simulink model "banc_essai_non_lineaire"  (R2021a)
settings: Solver=ode45  StartTime=0.0  StopTime=tfin  FixedStep=0.001  RelTol=1e-09  EnableMultiTasking=on
values from neighbouring files (symbols this model uses):
  Pzeq = .015    (= 0.015)    [main_non_lineaire.m]
undefined symbols (not defined in the file or in its folder): ae0, ae1, ae2, ae3, as0, as1, as2, as3, be1, g, Jx, Jy, LA, LB, LC, mSeff, mSg, mtot, RA, RB, RC, Vmax, XA, XB, XC, XD, XE, XF, YA, YB, YC, YD, YE, YF
settings Model: PacingRate=0.160000  Creator=delafontaine  LastModifiedBy=User
settings SolverCC: AlgebraicLoopSolver=LineSearch
settings DataIOCC: LimitDataPoints=on  SaveFormat=Array  SignalLoggingSaveFormat=ModelDataLogs  ReturnWorkspaceOutputs=off
settings OptimizationCC: LifeSpan=inf
settings DebuggingCC: UnderspecifiedInitializationDetection=Classic  MergeDetectMultiDrivingBlocksExec=none  MultiTaskDSMMsg=warning  MultiTaskCondExecSysMsg=none  SFUnexpectedBacktrackingDiag=warning  SFNoUnconditionalDefaultTransitionDiag=warning  SFExecutionAtInitializationDiag=none  SFMachineParentedDataDiag=warning  ArithmeticOperatorsInVariantConditions=warning
settings HardwareCC: ProdBitPerPointer=32  ProdBitPerSizeT=32  ProdBitPerPtrDiffT=32  ProdLargestAtomicFloat=None  ProdIntDivRoundTo=Undefined  ProdEndianess=Unspecified  ProdWordSize=32  ProdHWDeviceType=32-bit Generic
settings ModelReferenceCC: PropagateSignalLabelsOutOfModel=off
settings SFSimCC: SimUseLocalCustomCode=off  CustomCodeUndefinedFunction=UseInterfaceOnly
settings RTWCC: RTWUseLocalCustomCode=off
settings CodeAppCC: StateflowObjectComments=on
settings GRTTargetCC: TargetLangStandard=C89/C90 (ANSI)
settings ConfigComp: CovMetricSettings=dw  CovSaveCumulativeToWorkspaceVar=on  CovSaveSingleToWorkspaceVar=on  CovExternalEMLEnable=off  CovSFcnEnable=off

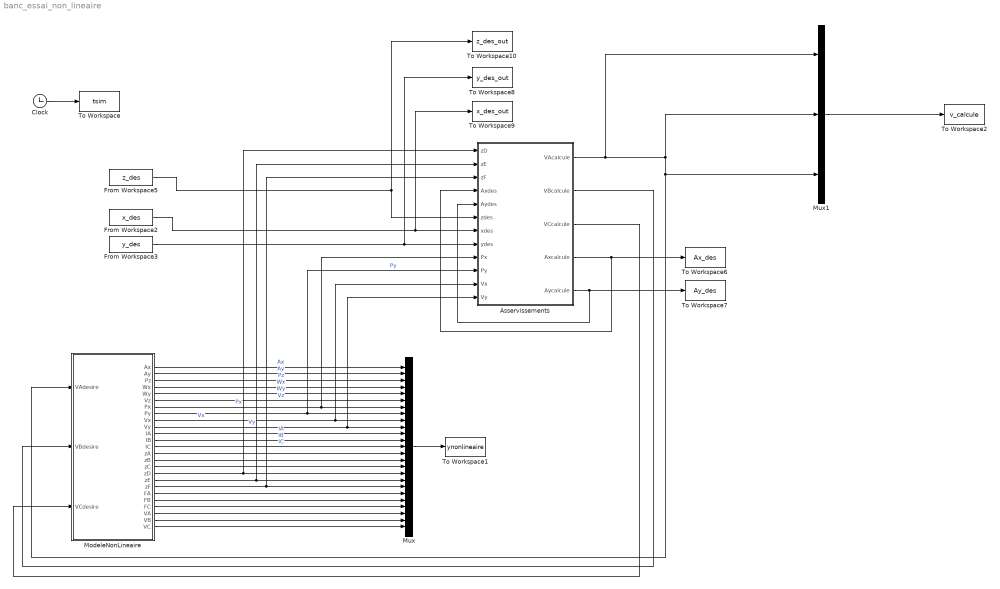
== system banc_essai_non_lineaire ==
  Asservissements : Subsystem
      mask help: Simulink:masks:GenSFuncDesc_MD
      mask Help: eval('feval(''rtwprivate'',''rtwhelpview'',''rtw_sfcn_block'')');
  Clock : Clock
  From Workspace2 : FromWorkspace  VariableName=x_des  Interpolate=off  OutputAfterFinalValue=Holding final value
  From Workspace3 : FromWorkspace  VariableName=y_des  Interpolate=off  OutputAfterFinalValue=Holding final value
  From Workspace5 : FromWorkspace  VariableName=z_des  Interpolate=off  OutputAfterFinalValue=Holding final value
  ModeleNonLineaire : Subsystem
      mask help: Simulink:masks:GenSFuncDesc_MD
      mask Help: eval('feval(''rtwprivate'',''rtwhelpview'',''rtw_sfcn_block'')');
  Mux : Mux  Inputs=25
  Mux1 : Mux  Inputs=3
  To Workspace : ToWorkspace  VariableName=tsim  SampleTime=-1
  To Workspace1 : ToWorkspace  VariableName=ynonlineaire  SampleTime=-1
  To Workspace10 : ToWorkspace  VariableName=z_des_out  SampleTime=-1
  To Workspace2 : ToWorkspace  VariableName=v_calcule  SampleTime=-1
  To Workspace6 : ToWorkspace  VariableName=Ax_des  SampleTime=-1
  To Workspace7 : ToWorkspace  VariableName=Ay_des  SampleTime=-1
  To Workspace8 : ToWorkspace  VariableName=y_des_out  SampleTime=-1
  To Workspace9 : ToWorkspace  VariableName=x_des_out  SampleTime=-1
  wires:
  Mux/1 -> To Workspace1/1
  Clock/1 -> To Workspace/1
  From Workspace5/1 -> Asservissements/6(zdes), To Workspace10/1
  ModeleNonLineaire/1(Ax) -> Mux/1  "Ax"
  ModeleNonLineaire/2(Ay) -> Mux/2  "Ay"
  ModeleNonLineaire/3(Pz) -> Mux/3  "Pz"
  ModeleNonLineaire/4(Wx) -> Mux/4  "Wx"
  ModeleNonLineaire/5(Wy) -> Mux/5  "Wy"
  ModeleNonLineaire/6(Vz) -> Mux/6  "Vz"
  ModeleNonLineaire/7(Px) -> Asservissements/9(Px), Mux/7  "Px"
  ModeleNonLineaire/8(Py) -> Asservissements/10(Py), Mux/8  "Py"
  ModeleNonLineaire/9(Vx) -> Asservissements/11(Vx), Mux/9  "Vx"
  ModeleNonLineaire/10(Vy) -> Asservissements/12(Vy), Mux/10  "Vy"
  ModeleNonLineaire/11(IA) -> Mux/11  "IA"
  ModeleNonLineaire/12(IB) -> Mux/12  "IB"
  ModeleNonLineaire/13(IC) -> Mux/13  "IC"
  From Workspace3/1 -> Asservissements/8(ydes), To Workspace8/1
  From Workspace2/1 -> Asservissements/7(xdes), To Workspace9/1
  ModeleNonLineaire/20(FA) -> Mux/20
  ModeleNonLineaire/21(FB) -> Mux/21
  ModeleNonLineaire/22(FC) -> Mux/22
  ModeleNonLineaire/23(VA) -> Mux/23
  ModeleNonLineaire/24(VB) -> Mux/24
  ModeleNonLineaire/25(VC) -> Mux/25
  Asservissements/4(Axcalcule) -> Asservissements/4(Axdes), To Workspace6/1
  Asservissements/5(Aycalcule) -> Asservissements/5(Aydes), To Workspace7/1
  Asservissements/1(VAcalcule) -> Mux1/1, Mux1/2, ModeleNonLineaire/1(VAdesire), Mux1/3
  Asservissements/2(VBcalcule) -> ModeleNonLineaire/2(VBdesire)
  Asservissements/3(VCcalcule) -> ModeleNonLineaire/3(VCdesire)
  ModeleNonLineaire/16(zC) -> Mux/16
  ModeleNonLineaire/17(zD) -> Asservissements/1(zD), Mux/17
  ModeleNonLineaire/18(zE) -> Asservissements/2(zE), Mux/18
  ModeleNonLineaire/19(zF) -> Asservissements/3(zF), Mux/19
  ModeleNonLineaire/14(zA) -> Mux/14
  ModeleNonLineaire/15(zB) -> Mux/15
  Mux1/1 -> To Workspace2/1

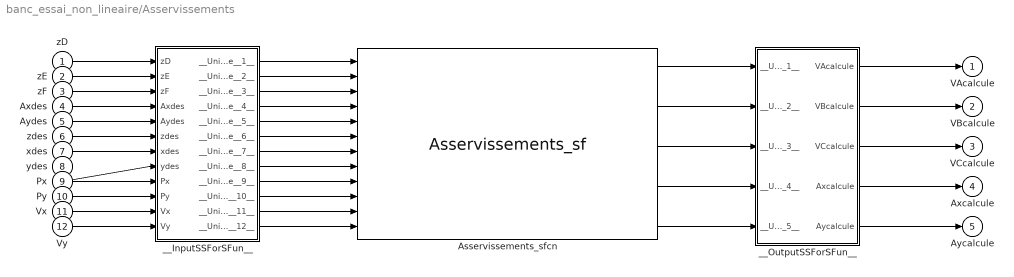
== system banc_essai_non_lineaire/Asservissements ==
  zD : Inport
  zE : Inport  Port=2
  zF : Inport  Port=3
  Axdes : Inport  Port=4
  Aydes : Inport  Port=5
  zdes : Inport  Port=6
  xdes : Inport  Port=7
  ydes : Inport  Port=8
  Px : Inport  Port=9
  Py : Inport  Port=10
  Vx : Inport  Port=11
  Vy : Inport  Port=12
  Asservissements_sfcn : S-Function  FunctionName=Asservissements_sf  SFunctionModules=""  SFunctionDeploymentMode=off  EnableBusSupport=off  mask{rtw_sf_name=Asservissements_sf, showVar=off}
      mask prompts: rtw_sf_name "Simulink:masks:GenSFuncName_MP"; showVar "Simulink:masks:GenSFuncShowModuleList_MP"
      mask help: Simulink:masks:GenSFuncDesc_MD
      mask init:
      | displist = '';
      | if ~strcmp(get_param(gcb, 'FunctionName'), rtw_sf_name);
      |   set_param(gcb, 'FunctionName', rtw_sf_name);
      | end
      | % Check if we are generating code
      | rtw_mode = false;
      | if strcmpi(get_param(bdroot(gcb),'SimulationStatus'),'Initializing')
      | 	rtw_mode = strcmpi(get_param(bdroot(gcb),'BuildingRTWCode'),'on') && ...
      | 		~strcmpi(get_param(bdroot(gcb),'TargetStyle'),'SimulationTarget');
      | end
      | if showVar || rtw_mode
      | 	if exist('rtwsfunc') == 2 | exist('rtwsfunc') == 6
      | 		tmplist = rtwsfunc(rtw_sf_name,gcb);
      | 		tmplist = DAStudio.message('Simulink:masks:GenSFuncListOfModules_IC', tmplist);
      | 	elseif showVar
      | 		tmplist1 = DAStudio.message('Simulink:masks:GenSFuncListOfModules_IC', '');
      |         tmplist2 = DAStudio.message('Simulink:masks:GenSFuncNotLicensed_IC');
      |         tmplist = [tmplist1 tmplist2];
      |  	end
      | end
      | if showVar
      |   displist = tmplist;
      | end
      settings: CopyFcn=|
      | if ~strcmp(get_param(gcb,'Linkstatus'),'none') && ...
      | ~strcmp(get_param(gcb,'Linkstatus'),'implicit')
      |   set_param(gcb,'LinkStatus','none');
      | end
      mask Help: eval('feval(''rtwprivate'',''rtwhelpview'',''rtw_sfcn_block'')');
      mask Display:
      | port_label('input',1,'zD');
      | port_label('input',2,'zE');
      | port_label('input',3,'zF');
      | port_label('input',4,'Axdes');
      | port_label('input',5,'Aydes');
      | port_label('input',6,'zdes');
      | port_label('input',7,'xdes');
      | port_label('input',8,'ydes');
      | port_label('input',9,'Px');
      | port_label('input',10,'Py');
      | port_label('input',11,'Vx');
      | port_label('input',12,'Vy');
      | port_label('output',1,'VAcalcule');
      | port_label('output',2,'VBcalcule');
      | port_label('output',3,'VCcalcule');
      | port_label('output',4,'Axcalcule');
      | port_label('output',5,'Aycalcule');
  __InputSSForSFun__ : Subsystem
  __OutputSSForSFun__ : Subsystem
  VAcalcule : Outport
  VBcalcule : Outport  Port=2
  VCcalcule : Outport  Port=3
  Axcalcule : Outport  Port=4
  Aycalcule : Outport  Port=5
  wires:
  zD/1 -> __InputSSForSFun__/1(zD)
  zE/1 -> __InputSSForSFun__/2(zE)
  zF/1 -> __InputSSForSFun__/3(zF)
  Axdes/1 -> __InputSSForSFun__/4(Axdes)
  Aydes/1 -> __InputSSForSFun__/5(Aydes)
  zdes/1 -> __InputSSForSFun__/6(zdes)
  xdes/1 -> __InputSSForSFun__/7(xdes)
  ydes/1 -> __InputSSForSFun__/8(ydes)
  Px/1 -> __InputSSForSFun__/9(Px)
  Py/1 -> __InputSSForSFun__/10(Py)
  Vx/1 -> __InputSSForSFun__/11(Vx)
  Vy/1 -> __InputSSForSFun__/12(Vy)
  __InputSSForSFun__/1(__UniqueOutportName__1__) -> Asservissements_sfcn/1
  __InputSSForSFun__/2(__UniqueOutportName__2__) -> Asservissements_sfcn/2
  __InputSSForSFun__/3(__UniqueOutportName__3__) -> Asservissements_sfcn/3
  __InputSSForSFun__/4(__UniqueOutportName__4__) -> Asservissements_sfcn/4
  __InputSSForSFun__/5(__UniqueOutportName__5__) -> Asservissements_sfcn/5
  __InputSSForSFun__/6(__UniqueOutportName__6__) -> Asservissements_sfcn/6
  __InputSSForSFun__/7(__UniqueOutportName__7__) -> Asservissements_sfcn/7
  __InputSSForSFun__/8(__UniqueOutportName__8__) -> Asservissements_sfcn/8
  __InputSSForSFun__/9(__UniqueOutportName__9__) -> Asservissements_sfcn/9
  __InputSSForSFun__/10(__UniqueOutportName__10__) -> Asservissements_sfcn/10
  __InputSSForSFun__/11(__UniqueOutportName__11__) -> Asservissements_sfcn/11
  __InputSSForSFun__/12(__UniqueOutportName__12__) -> Asservissements_sfcn/12
  Asservissements_sfcn/1 -> __OutputSSForSFun__/1(__UniqueInportName__1__)
  Asservissements_sfcn/2 -> __OutputSSForSFun__/2(__UniqueInportName__2__)
  Asservissements_sfcn/3 -> __OutputSSForSFun__/3(__UniqueInportName__3__)
  Asservissements_sfcn/4 -> __OutputSSForSFun__/4(__UniqueInportName__4__)
  Asservissements_sfcn/5 -> __OutputSSForSFun__/5(__UniqueInportName__5__)
  __OutputSSForSFun__/1(VAcalcule) -> VAcalcule/1
  __OutputSSForSFun__/2(VBcalcule) -> VBcalcule/1
  __OutputSSForSFun__/3(VCcalcule) -> VCcalcule/1
  __OutputSSForSFun__/4(Axcalcule) -> Axcalcule/1
  __OutputSSForSFun__/5(Aycalcule) -> Aycalcule/1

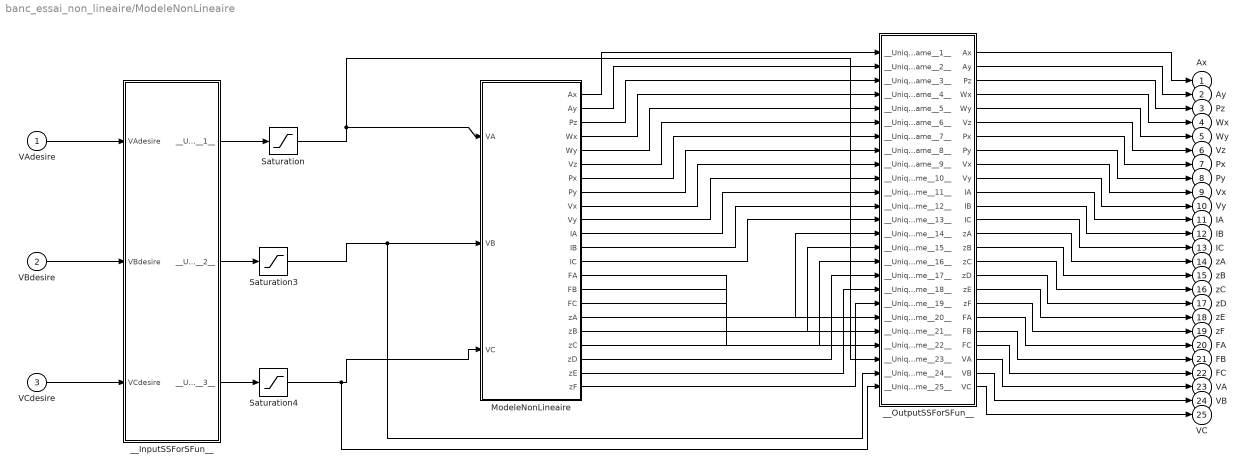
== system banc_essai_non_lineaire/ModeleNonLineaire ==
  VAdesire : Inport
  VBdesire : Inport  Port=2
  VCdesire : Inport  Port=3
  ModeleNonLineaire : Subsystem
  Saturation : Saturate  UpperLimit=0  LowerLimit=-Vmax
  Saturation3 : Saturate  UpperLimit=0  LowerLimit=-Vmax
  Saturation4 : Saturate  UpperLimit=0  LowerLimit=-Vmax
  __InputSSForSFun__ : Subsystem
  __OutputSSForSFun__ : Subsystem
  Ax : Outport
  Ay : Outport  Port=2
  Pz : Outport  Port=3
  Wx : Outport  Port=4
  Wy : Outport  Port=5
  Vz : Outport  Port=6
  Px : Outport  Port=7
  Py : Outport  Port=8
  Vx : Outport  Port=9
  Vy : Outport  Port=10
  IA : Outport  Port=11
  IB : Outport  Port=12
  IC : Outport  Port=13
  zA : Outport  Port=14
  zB : Outport  Port=15
  zC : Outport  Port=16
  zD : Outport  Port=17
  zE : Outport  Port=18
  zF : Outport  Port=19
  FA : Outport  Port=20
  FB : Outport  Port=21
  FC : Outport  Port=22
  VA : Outport  Port=23
  VB : Outport  Port=24
  VC : Outport  Port=25
  wires:
  VAdesire/1 -> __InputSSForSFun__/1(VAdesire)
  VBdesire/1 -> __InputSSForSFun__/2(VBdesire)
  VCdesire/1 -> __InputSSForSFun__/3(VCdesire)
  __InputSSForSFun__/2(__UniqueOutportName__2__) -> Saturation3/1
  __InputSSForSFun__/3(__UniqueOutportName__3__) -> Saturation4/1
  ModeleNonLineaire/1(Ax) -> __OutputSSForSFun__/1(__UniqueInportName__1__)
  ModeleNonLineaire/2(Ay) -> __OutputSSForSFun__/2(__UniqueInportName__2__)
  ModeleNonLineaire/3(Pz) -> __OutputSSForSFun__/3(__UniqueInportName__3__)
  ModeleNonLineaire/4(Wx) -> __OutputSSForSFun__/4(__UniqueInportName__4__)
  ModeleNonLineaire/5(Wy) -> __OutputSSForSFun__/5(__UniqueInportName__5__)
  ModeleNonLineaire/6(Vz) -> __OutputSSForSFun__/6(__UniqueInportName__6__)
  ModeleNonLineaire/7(Px) -> __OutputSSForSFun__/7(__UniqueInportName__7__)
  ModeleNonLineaire/8(Py) -> __OutputSSForSFun__/8(__UniqueInportName__8__)
  ModeleNonLineaire/9(Vx) -> __OutputSSForSFun__/9(__UniqueInportName__9__)
  ModeleNonLineaire/10(Vy) -> __OutputSSForSFun__/10(__UniqueInportName__10__)
  ModeleNonLineaire/11(IA) -> __OutputSSForSFun__/11(__UniqueInportName__11__)
  ModeleNonLineaire/12(IB) -> __OutputSSForSFun__/12(__UniqueInportName__12__)
  ModeleNonLineaire/13(IC) -> __OutputSSForSFun__/13(__UniqueInportName__13__)
  __OutputSSForSFun__/1(Ax) -> Ax/1
  __OutputSSForSFun__/2(Ay) -> Ay/1
  __OutputSSForSFun__/3(Pz) -> Pz/1
  __OutputSSForSFun__/4(Wx) -> Wx/1
  __OutputSSForSFun__/5(Wy) -> Wy/1
  __OutputSSForSFun__/6(Vz) -> Vz/1
  __OutputSSForSFun__/7(Px) -> Px/1
  __OutputSSForSFun__/8(Py) -> Py/1
  __OutputSSForSFun__/9(Vx) -> Vx/1
  __OutputSSForSFun__/10(Vy) -> Vy/1
  __OutputSSForSFun__/11(IA) -> IA/1
  __OutputSSForSFun__/12(IB) -> IB/1
  __OutputSSForSFun__/13(IC) -> IC/1
  __OutputSSForSFun__/14(zA) -> zA/1
  __OutputSSForSFun__/15(zB) -> zB/1
  __OutputSSForSFun__/16(zC) -> zC/1
  __OutputSSForSFun__/17(zD) -> zD/1
  __OutputSSForSFun__/18(zE) -> zE/1
  __OutputSSForSFun__/19(zF) -> zF/1
  __OutputSSForSFun__/20(FA) -> FA/1
  __OutputSSForSFun__/21(FB) -> FB/1
  __OutputSSForSFun__/22(FC) -> FC/1
  __OutputSSForSFun__/23(VA) -> VA/1
  __OutputSSForSFun__/24(VB) -> VB/1
  __OutputSSForSFun__/25(VC) -> VC/1
  ModeleNonLineaire/14(FA) -> __OutputSSForSFun__/20(__UniqueInportName__20__)
  ModeleNonLineaire/15(FB) -> __OutputSSForSFun__/21(__UniqueInportName__21__)
  ModeleNonLineaire/16(FC) -> __OutputSSForSFun__/22(__UniqueInportName__22__)
  ModeleNonLineaire/17(zA) -> __OutputSSForSFun__/14(__UniqueInportName__14__)
  ModeleNonLineaire/18(zB) -> __OutputSSForSFun__/15(__UniqueInportName__15__)
  ModeleNonLineaire/19(zC) -> __OutputSSForSFun__/16(__UniqueInportName__16__)
  ModeleNonLineaire/20(zD) -> __OutputSSForSFun__/17(__UniqueInportName__17__)
  ModeleNonLineaire/21(zE) -> __OutputSSForSFun__/18(__UniqueInportName__18__)
  ModeleNonLineaire/22(zF) -> __OutputSSForSFun__/19(__UniqueInportName__19__)
  __InputSSForSFun__/1(__UniqueOutportName__1__) -> Saturation/1
  Saturation3/1 -> ModeleNonLineaire/2(VB), __OutputSSForSFun__/24(__UniqueInportName__24__)
  Saturation4/1 -> ModeleNonLineaire/3(VC), __OutputSSForSFun__/25(__UniqueInportName__25__)
  Saturation/1 -> ModeleNonLineaire/1(VA), __OutputSSForSFun__/23(__UniqueInportName__23__)

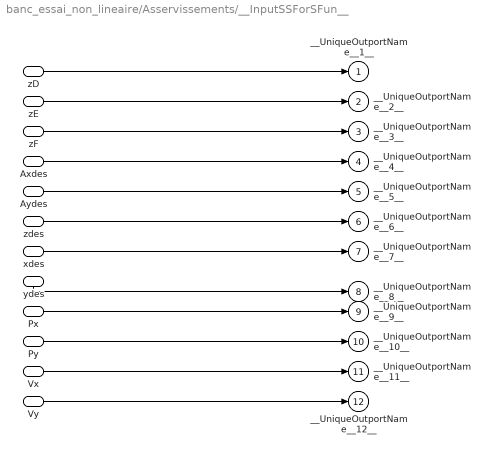
== system banc_essai_non_lineaire/Asservissements/__InputSSForSFun__ ==
  zD : Inport
  zE : Inport  Port=2
  zF : Inport  Port=3
  Axdes : Inport  Port=4
  Aydes : Inport  Port=5
  zdes : Inport  Port=6
  xdes : Inport  Port=7
  ydes : Inport  Port=8
  Px : Inport  Port=9
  Py : Inport  Port=10
  Vx : Inport  Port=11
  Vy : Inport  Port=12
  __UniqueOutportName__1__ : Outport
  __UniqueOutportName__2__ : Outport  Port=2
  __UniqueOutportName__3__ : Outport  Port=3
  __UniqueOutportName__4__ : Outport  Port=4
  __UniqueOutportName__5__ : Outport  Port=5
  __UniqueOutportName__6__ : Outport  Port=6
  __UniqueOutportName__7__ : Outport  Port=7
  __UniqueOutportName__8__ : Outport  Port=8
  __UniqueOutportName__9__ : Outport  Port=9
  __UniqueOutportName__10__ : Outport  Port=10
  __UniqueOutportName__11__ : Outport  Port=11
  __UniqueOutportName__12__ : Outport  Port=12
  wires:
  zD/1 -> __UniqueOutportName__1__/1
  zE/1 -> __UniqueOutportName__2__/1
  zF/1 -> __UniqueOutportName__3__/1
  Axdes/1 -> __UniqueOutportName__4__/1
  Aydes/1 -> __UniqueOutportName__5__/1
  zdes/1 -> __UniqueOutportName__6__/1
  xdes/1 -> __UniqueOutportName__7__/1
  ydes/1 -> __UniqueOutportName__8__/1
  Px/1 -> __UniqueOutportName__9__/1
  Py/1 -> __UniqueOutportName__10__/1
  Vx/1 -> __UniqueOutportName__11__/1
  Vy/1 -> __UniqueOutportName__12__/1

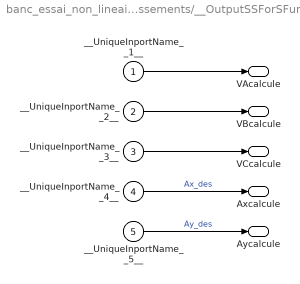
== system banc_essai_non_lineaire/Asservissements/__OutputSSForSFun__ ==
  __UniqueInportName__1__ : Inport
  __UniqueInportName__2__ : Inport  Port=2
  __UniqueInportName__3__ : Inport  Port=3
  __UniqueInportName__4__ : Inport  Port=4
  __UniqueInportName__5__ : Inport  Port=5
  VAcalcule : Outport
  VBcalcule : Outport  Port=2
  VCcalcule : Outport  Port=3
  Axcalcule : Outport  Port=4
  Aycalcule : Outport  Port=5
  wires:
  __UniqueInportName__1__/1 -> VAcalcule/1
  __UniqueInportName__2__/1 -> VBcalcule/1
  __UniqueInportName__3__/1 -> VCcalcule/1
  __UniqueInportName__4__/1 -> Axcalcule/1  "Ax_des"
  __UniqueInportName__5__/1 -> Aycalcule/1  "Ay_des"

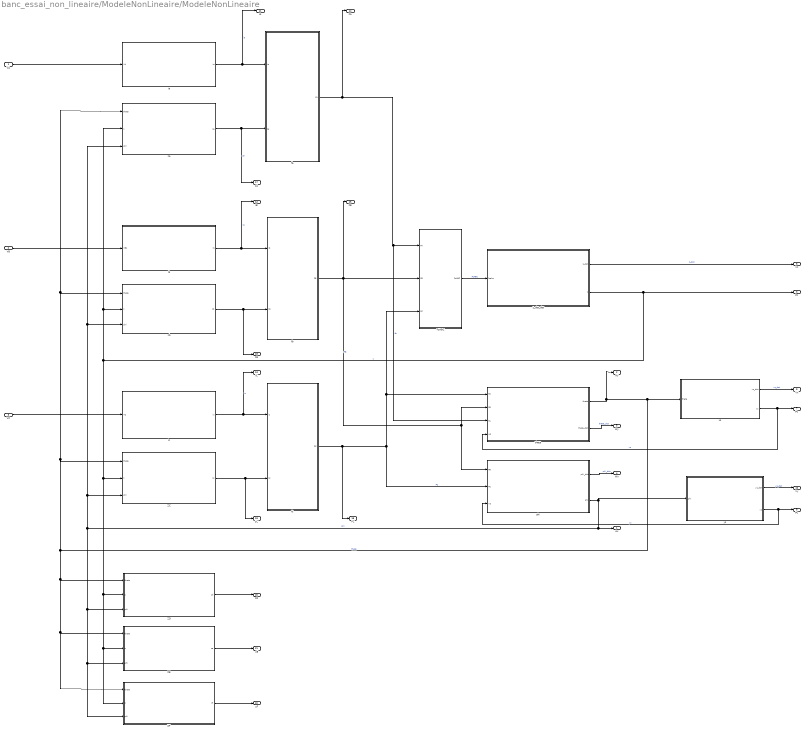
== system banc_essai_non_lineaire/ModeleNonLineaire/ModeleNonLineaire ==
  VA : Inport
  VB : Inport  Port=2
  VC : Inport  Port=3
  FzABC : Subsystem
  ZC : Subsystem
  ZD : Subsystem
  ZE : Subsystem
  ZF : Subsystem
  fa : Subsystem
  fb : Subsystem
  fc : Subsystem
  ia : Subsystem
  ib : Subsystem
  ic : Subsystem
  phi : Subsystem
  theta : Subsystem
  xs : Subsystem
  ys : Subsystem
  z_dot_dot : Subsystem
  za : Subsystem
  zb : Subsystem
  Ax : Outport
  Ay : Outport  Port=2
  Pz : Outport  Port=3
  Wx : Outport  Port=4
  Wy : Outport  Port=5
  Vz : Outport  Port=6
  Px : Outport  Port=7
  Py : Outport  Port=8
  Vx : Outport  Port=9
  Vy : Outport  Port=10
  IA : Outport  Port=11
  IB : Outport  Port=12
  IC : Outport  Port=13
  FA : Outport  Port=14
  FB : Outport  Port=15
  FC : Outport  Port=16
  zA : Outport  Port=17
  zB : Outport  Port=18
  zC : Outport  Port=19
  zD : Outport  Port=20
  zE : Outport  Port=21
  zF : Outport  Port=22
  wires:
  ia/1(ia) -> fa/1(ia), IA/1  "ia"
  ic/1(ic) -> IC/1, fc/1(ic)  "ic"
  phi/2(phi) -> ys/1(phi), Ax/1, za/3(phi), zb/3(phi), ZC/3(phi), ZD/3(phi), ZF/3(phi), ZE/3(phi)  "phi"
  theta/1(theta) -> xs/1(theta), ZD/1(theta), ZF/1(theta), ZE/1(theta), za/1(theta), zb/1(theta), ZC/1(theta), Ay/1  "theta"
  fa/1(FA) -> theta/3(FA), FzABC/1(FA), FA/1  "fa"
  fb/1(FB) -> FzABC/2(FB), phi/1(FB), theta/2(FB), FB/1  "FB"
  fc/1(FC) -> FC/1, phi/2(FC), FzABC/3(FC), theta/1(FC)  "FC"
  ZC/1(zc) -> zC/1, fc/2(zc)
  zb/1(zb) -> zB/1, fb/2(zb)
  ib/1(ib) -> fb/1(ib), IB/1  "ib"
  FzABC/1(FzABC) -> z_dot_dot/1(fzabc)  "FzABC"
  za/1(za) -> zA/1, fa/2(za)  "za"
  theta/2(theta_dot) -> Wy/1  "theta_dot"
  xs/1(xs_dot) -> Vx/1  "xs_dot"
  z_dot_dot/2(z) -> za/2(z), zb/2(z), ZD/2(z), ZF/2(z), ZE/2(z), ZC/2(z), Pz/1  "z"
  phi/1(phi_dot) -> Wx/1  "phi_dot"
  ys/2(ys) -> phi/3(YS), Py/1  "ys"
  VB/1 -> ib/1(VB1)
  z_dot_dot/1(z_dot) -> Vz/1  "z_dot"
  xs/2(xs) -> theta/4(XS), Px/1  "xs"
  ys/1(ys_dot) -> Vy/1  "ys_dot"
  VA/1 -> ia/1(VA)
  VC/1 -> ic/1(VC)
  ZD/1(zd) -> zD/1
  ZF/1(zf) -> zF/1
  ZE/1(ze) -> zE/1

== system banc_essai_non_lineaire/ModeleNonLineaire/__InputSSForSFun__ ==
  VAdesire : Inport
  VBdesire : Inport  Port=2
  VCdesire : Inport  Port=3
  __UniqueOutportName__1__ : Outport
  __UniqueOutportName__2__ : Outport  Port=2
  __UniqueOutportName__3__ : Outport  Port=3
  wires:
  VAdesire/1 -> __UniqueOutportName__1__/1
  VBdesire/1 -> __UniqueOutportName__2__/1
  VCdesire/1 -> __UniqueOutportName__3__/1

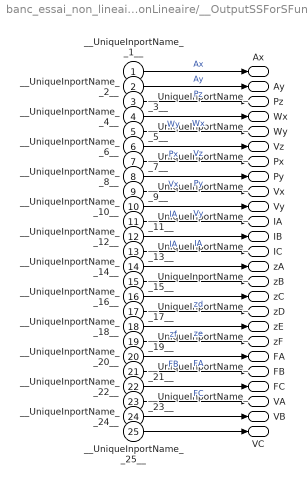
== system banc_essai_non_lineaire/ModeleNonLineaire/__OutputSSForSFun__ ==
  __UniqueInportName__1__ : Inport
  __UniqueInportName__2__ : Inport  Port=2
  __UniqueInportName__3__ : Inport  Port=3
  __UniqueInportName__4__ : Inport  Port=4
  __UniqueInportName__5__ : Inport  Port=5
  __UniqueInportName__6__ : Inport  Port=6
  __UniqueInportName__7__ : Inport  Port=7
  __UniqueInportName__8__ : Inport  Port=8
  __UniqueInportName__9__ : Inport  Port=9
  __UniqueInportName__10__ : Inport  Port=10
  __UniqueInportName__11__ : Inport  Port=11
  __UniqueInportName__12__ : Inport  Port=12
  __UniqueInportName__13__ : Inport  Port=13
  __UniqueInportName__14__ : Inport  Port=14
  __UniqueInportName__15__ : Inport  Port=15
  __UniqueInportName__16__ : Inport  Port=16
  __UniqueInportName__17__ : Inport  Port=17
  __UniqueInportName__18__ : Inport  Port=18
  __UniqueInportName__19__ : Inport  Port=19
  __UniqueInportName__20__ : Inport  Port=20
  __UniqueInportName__21__ : Inport  Port=21
  __UniqueInportName__22__ : Inport  Port=22
  __UniqueInportName__23__ : Inport  Port=23
  __UniqueInportName__24__ : Inport  Port=24
  __UniqueInportName__25__ : Inport  Port=25
  Ax : Outport
  Ay : Outport  Port=2
  Pz : Outport  Port=3
  Wx : Outport  Port=4
  Wy : Outport  Port=5
  Vz : Outport  Port=6
  Px : Outport  Port=7
  Py : Outport  Port=8
  Vx : Outport  Port=9
  Vy : Outport  Port=10
  IA : Outport  Port=11
  IB : Outport  Port=12
  IC : Outport  Port=13
  zA : Outport  Port=14
  zB : Outport  Port=15
  zC : Outport  Port=16
  zD : Outport  Port=17
  zE : Outport  Port=18
  zF : Outport  Port=19
  FA : Outport  Port=20
  FB : Outport  Port=21
  FC : Outport  Port=22
  VA : Outport  Port=23
  VB : Outport  Port=24
  VC : Outport  Port=25
  wires:
  __UniqueInportName__1__/1 -> Ax/1  "Ax"
  __UniqueInportName__2__/1 -> Ay/1  "Ay"
  __UniqueInportName__3__/1 -> Pz/1  "Pz"
  __UniqueInportName__4__/1 -> Wx/1  "Wx"
  __UniqueInportName__5__/1 -> Wy/1  "Wy"
  __UniqueInportName__6__/1 -> Vz/1  "Vz"
  __UniqueInportName__7__/1 -> Px/1  "Px"
  __UniqueInportName__8__/1 -> Py/1  "Py"
  __UniqueInportName__9__/1 -> Vx/1  "Vx"
  __UniqueInportName__10__/1 -> Vy/1  "Vy"
  __UniqueInportName__11__/1 -> IA/1  "IA"
  __UniqueInportName__12__/1 -> IB/1  "IA"
  __UniqueInportName__13__/1 -> IC/1  "IA"
  __UniqueInportName__14__/1 -> zA/1
  __UniqueInportName__15__/1 -> zB/1
  __UniqueInportName__16__/1 -> zC/1
  __UniqueInportName__17__/1 -> zD/1  "zd"
  __UniqueInportName__18__/1 -> zE/1  "ze"
  __UniqueInportName__19__/1 -> zF/1  "zf"
  __UniqueInportName__20__/1 -> FA/1  "FA"
  __UniqueInportName__21__/1 -> FB/1  "FB"
  __UniqueInportName__22__/1 -> FC/1  "FC"
  __UniqueInportName__23__/1 -> VA/1
  __UniqueInportName__24__/1 -> VB/1
  __UniqueInportName__25__/1 -> VC/1

== system banc_essai_non_lineaire/ModeleNonLineaire/ModeleNonLineaire/FzABC ==
  FA : Inport
  FB : Inport  Port=2
  FC : Inport  Port=3
  Sum of Elements1 : Sum  Inputs=+++
  FzABC : Outport
  wires:
  FC/1 -> Sum of Elements1/3
  Sum of Elements1/1 -> FzABC/1  "FzABC"
  FA/1 -> Sum of Elements1/1
  FB/1 -> Sum of Elements1/2

== system banc_essai_non_lineaire/ModeleNonLineaire/ModeleNonLineaire/ZC ==
  theta : Inport
  z : Inport  Port=2
  phi : Inport  Port=3
  Constant2 : Constant  Value=-XC
  Constant3 : Constant  Value=YC
  Product2 : Product
  Product3 : Product
  Sum5 : Sum  Inputs=|+++
  zc : Outport
  wires:
  Constant2/1 -> Product2/2
  z/1 -> Sum5/1
  Constant3/1 -> Product3/1
  Product3/1 -> Sum5/3
  Sum5/1 -> zc/1  "zc"
  Product2/1 -> Sum5/2
  phi/1 -> Product3/2
  theta/1 -> Product2/1

== system banc_essai_non_lineaire/ModeleNonLineaire/ModeleNonLineaire/ZD ==
  theta : Inport
  z : Inport  Port=2
  phi : Inport  Port=3
  Constant2 : Constant  Value=-XD
  Constant3 : Constant  Value=YD
  Product2 : Product
  Product3 : Product
  Sum5 : Sum  Inputs=|+++
  zd : Outport
  wires:
  Product2/1 -> Sum5/2
  Constant3/1 -> Product3/1
  Constant2/1 -> Product2/2
  z/1 -> Sum5/1
  Product3/1 -> Sum5/3
  Sum5/1 -> zd/1  "zd"
  theta/1 -> Product2/1
  phi/1 -> Product3/2

== system banc_essai_non_lineaire/ModeleNonLineaire/ModeleNonLineaire/ZE ==
  theta : Inport
  z : Inport  Port=2
  phi : Inport  Port=3
  Constant2 : Constant  Value=-XE
  Constant3 : Constant  Value=YE
  Product2 : Product
  Product3 : Product
  Sum5 : Sum  Inputs=|+++
  ze : Outport
  wires:
  Product2/1 -> Sum5/2
  Constant3/1 -> Product3/1
  Constant2/1 -> Product2/2
  z/1 -> Sum5/1
  Product3/1 -> Sum5/3
  Sum5/1 -> ze/1  "ze"
  theta/1 -> Product2/1
  phi/1 -> Product3/2

== system banc_essai_non_lineaire/ModeleNonLineaire/ModeleNonLineaire/ZF ==
  theta : Inport
  z : Inport  Port=2
  phi : Inport  Port=3
  Constant2 : Constant  Value=-XF
  Constant3 : Constant  Value=YF
  Product2 : Product
  Product3 : Product
  Sum5 : Sum  Inputs=|+++
  zf : Outport
  wires:
  Product2/1 -> Sum5/2
  Constant3/1 -> Product3/1
  Constant2/1 -> Product2/2
  z/1 -> Sum5/1
  Product3/1 -> Sum5/3
  Sum5/1 -> zf/1  "zf"
  theta/1 -> Product2/1
  phi/1 -> Product3/2

== system banc_essai_non_lineaire/ModeleNonLineaire/ModeleNonLineaire/fa ==
  ia : Inport
  za : Inport  Port=2
  fa : Subsystem
  FA : Outport
  wires:
  za/1 -> fa/2(za)
  ia/1 -> fa/1(ia)
  fa/1(FA) -> FA/1

== system banc_essai_non_lineaire/ModeleNonLineaire/ModeleNonLineaire/fb ==
  ib : Inport
  zb : Inport  Port=2
  FB_num : Subsystem
  FB : Outport
  wires:
  zb/1 -> FB_num/2(zb)
  ib/1 -> FB_num/1(ib)
  FB_num/1(FB) -> FB/1

== system banc_essai_non_lineaire/ModeleNonLineaire/ModeleNonLineaire/fc ==
  ic : Inport
  zc : Inport  Port=2
  fc : Subsystem
  FC : Outport
  wires:
  zc/1 -> fc/2(zc)
  ic/1 -> fc/1(ic)
  fc/1(FC) -> FC/1

== system banc_essai_non_lineaire/ModeleNonLineaire/ModeleNonLineaire/ia ==
  VA : Inport
  Gain : Gain  Gain=-RA/LA
  Gain1 : Gain  Gain=1/LA
  Integrator : Integrator
  Sum : Sum  Inputs=|++
  ia : Outport
  wires:
  Sum/1 -> Integrator/1  "ia_dot"
  Integrator/1 -> ia/1, Gain/1  "ia"
  Gain1/1 -> Sum/2
  Gain/1 -> Sum/1
  VA/1 -> Gain1/1

== system banc_essai_non_lineaire/ModeleNonLineaire/ModeleNonLineaire/ib ==
  VB1 : Inport
  Gain2 : Gain  Gain=-RB/LB
  Gain3 : Gain  Gain=1/LB
  Integrator1 : Integrator
  Sum1 : Sum  Inputs=|++
  ib : Outport
  wires:
  Sum1/1 -> Integrator1/1  "ib_dot"
  VB1/1 -> Gain3/1
  Integrator1/1 -> ib/1, Gain2/1  "ib"
  Gain2/1 -> Sum1/1
  Gain3/1 -> Sum1/2

== system banc_essai_non_lineaire/ModeleNonLineaire/ModeleNonLineaire/ic ==
  VC : Inport
  Gain4 : Gain  Gain=-RC/LC
  Gain5 : Gain  Gain=1/LC
  Integrator2 : Integrator
  Sum2 : Sum  Inputs=|++
  ic : Outport
  wires:
  Integrator2/1 -> ic/1, Gain4/1  "ic"
  Gain5/1 -> Sum2/2
  Gain4/1 -> Sum2/1
  Sum2/1 -> Integrator2/1  "ic_dot"
  VC/1 -> Gain5/1

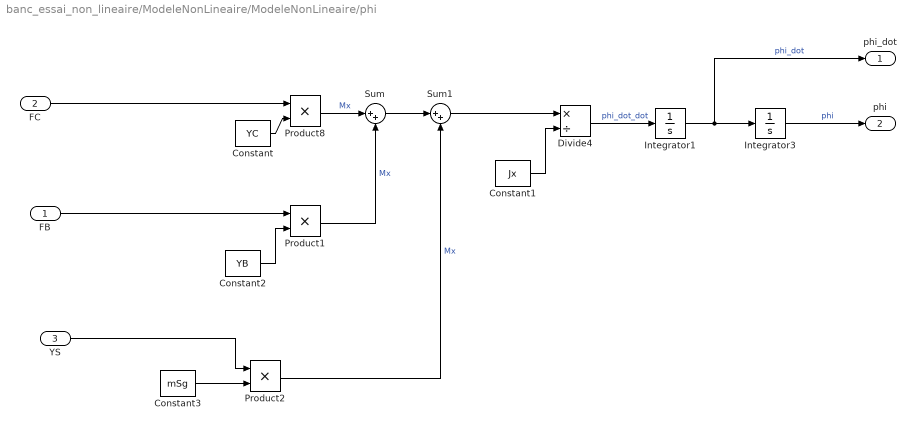
== system banc_essai_non_lineaire/ModeleNonLineaire/ModeleNonLineaire/phi ==
  FB : Inport
  FC : Inport  Port=2
  YS : Inport  Port=3
  Constant : Constant  Value=YC
  Constant1 : Constant  Value=Jx
  Constant2 : Constant  Value=YB
  Constant3 : Constant  Value=mSg
  Divide4 : Product  Inputs=*/
  Integrator1 : Integrator
  Integrator3 : Integrator
  Product1 : Product
  Product2 : Product
  Product8 : Product
  Sum : Sum  Inputs=|++
  Sum1 : Sum  Inputs=|++
  phi_dot : Outport
  phi : Outport  Port=2
  wires:
  FC/1 -> Product8/1
  Integrator3/1 -> phi/1  "phi"
  Constant/1 -> Product8/2
  Constant1/1 -> Divide4/2
  Integrator1/1 -> phi_dot/1, Integrator3/1  "phi_dot"
  Divide4/1 -> Integrator1/1  "phi_dot_dot"
  FB/1 -> Product1/1
  Constant2/1 -> Product1/2
  Product8/1 -> Sum/1  "Mx"
  Product1/1 -> Sum/2  "Mx"
  YS/1 -> Product2/1
  Constant3/1 -> Product2/2
  Sum/1 -> Sum1/1
  Sum1/1 -> Divide4/1
  Product2/1 -> Sum1/2  "Mx"

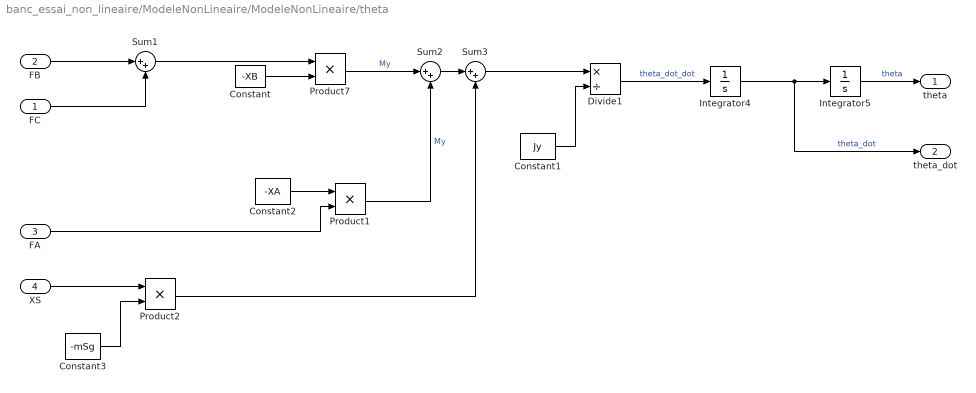
== system banc_essai_non_lineaire/ModeleNonLineaire/ModeleNonLineaire/theta ==
  FC : Inport
  FB : Inport  Port=2
  FA : Inport  Port=3
  XS : Inport  Port=4
  Constant : Constant  Value=-XB
  Constant1 : Constant  Value=Jy
  Constant2 : Constant  Value=-XA
  Constant3 : Constant  Value=-mSg
  Divide1 : Product  Inputs=*/
  Integrator4 : Integrator
  Integrator5 : Integrator
  Product1 : Product
  Product2 : Product
  Product7 : Product
  Sum1 : Sum  Inputs=|++
  Sum2 : Sum  Inputs=|++
  Sum3 : Sum  Inputs=|++
  theta : Outport
  theta_dot : Outport  Port=2
  wires:
  FB/1 -> Sum1/1
  FC/1 -> Sum1/2
  Constant1/1 -> Divide1/2
  Sum1/1 -> Product7/1
  Integrator4/1 -> theta_dot/1, Integrator5/1  "theta_dot"
  Product7/1 -> Sum2/1  "My"
  Constant/1 -> Product7/2
  Divide1/1 -> Integrator4/1  "theta_dot_dot"
  Integrator5/1 -> theta/1  "theta"
  Constant2/1 -> Product1/1
  FA/1 -> Product1/2
  Product1/1 -> Sum2/2  "My"
  XS/1 -> Product2/1
  Constant3/1 -> Product2/2
  Sum2/1 -> Sum3/1
  Sum3/1 -> Divide1/1
  Product2/1 -> Sum3/2

== system banc_essai_non_lineaire/ModeleNonLineaire/ModeleNonLineaire/xs ==
  theta : Inport
  Constant : Constant  Value=mSeff
  Constant1 : Constant  Value=-mSg
  Divide2 : Product  Inputs=*/
  Integrator : Integrator
  Integrator1 : Integrator
  Product : Product
  xs_dot : Outport
  xs : Outport  Port=2
  wires:
  Constant/1 -> Divide2/2
  Constant1/1 -> Divide2/1
  Divide2/1 -> Product/1
  theta/1 -> Product/2
  Product/1 -> Integrator/1  "xs_dot_dot"
  Integrator/1 -> Integrator1/1, xs_dot/1  "xs_dot"
  Integrator1/1 -> xs/1  "xs"

== system banc_essai_non_lineaire/ModeleNonLineaire/ModeleNonLineaire/ys ==
  phi : Inport
  Constant : Constant  Value=mSeff
  Constant1 : Constant  Value=mSg
  Divide1 : Product  Inputs=*/
  Integrator : Integrator
  Integrator1 : Integrator
  Product1 : Product
  ys_dot : Outport
  ys : Outport  Port=2
  wires:
  Constant/1 -> Divide1/2
  Divide1/1 -> Product1/1
  Constant1/1 -> Divide1/1
  phi/1 -> Product1/2
  Product1/1 -> Integrator/1  "ys_dot_dot"
  Integrator/1 -> Integrator1/1, ys_dot/1  "ys_dot"
  Integrator1/1 -> ys/1  "ys"

== system banc_essai_non_lineaire/ModeleNonLineaire/ModeleNonLineaire/z_dot_dot ==
  fzabc : Inport
  Constant1 : Constant  Value=mtot
  Constant2 : Constant  Value=g
  Divide3 : Product  Inputs=*/
  Integrator : Integrator  UpperSaturationLimit=0.05  LowerSaturationLimit=-0.05
  Integrator1 : Integrator  InitialCondition=Pzeq  LimitOutput=on  UpperSaturationLimit=30/1000  LowerSaturationLimit=0
  Sum9 : Sum  Inputs=|++
  z_dot : Outport
  z : Outport  Port=2
  wires:
  Constant1/1 -> Divide3/2
  Constant2/1 -> Sum9/2
  Divide3/1 -> Sum9/1
  fzabc/1 -> Divide3/1
  Sum9/1 -> Integrator/1  "z_dot_dot"
  Integrator/1 -> Integrator1/1, z_dot/1  "z_dot"
  Integrator1/1 -> z/1  "z"

== system banc_essai_non_lineaire/ModeleNonLineaire/ModeleNonLineaire/za ==
  theta : Inport
  z : Inport  Port=2
  phi : Inport  Port=3
  Constant1 : Constant  Value=-XA
  Constant2 : Constant  Value=YA
  Product2 : Product
  Product3 : Product
  Sum5 : Sum  Inputs=|+++
  za : Outport
  wires:
  z/1 -> Sum5/1
  Product3/1 -> Sum5/3
  Constant2/1 -> Product3/1
  Constant1/1 -> Product2/2
  Product2/1 -> Sum5/2
  Sum5/1 -> za/1  "za"
  phi/1 -> Product3/2
  theta/1 -> Product2/1

== system banc_essai_non_lineaire/ModeleNonLineaire/ModeleNonLineaire/zb ==
  theta : Inport
  z : Inport  Port=2
  phi : Inport  Port=3
  Constant : Constant  Value=-XB
  Constant1 : Constant  Value=YB
  Product2 : Product
  Product3 : Product
  Sum5 : Sum  Inputs=|+++
  zb : Outport
  wires:
  Constant1/1 -> Product3/1
  Constant/1 -> Product2/2
  Product3/1 -> Sum5/3
  Product2/1 -> Sum5/2
  Sum5/1 -> zb/1  "zb"
  z/1 -> Sum5/1
  theta/1 -> Product2/1
  phi/1 -> Product3/2

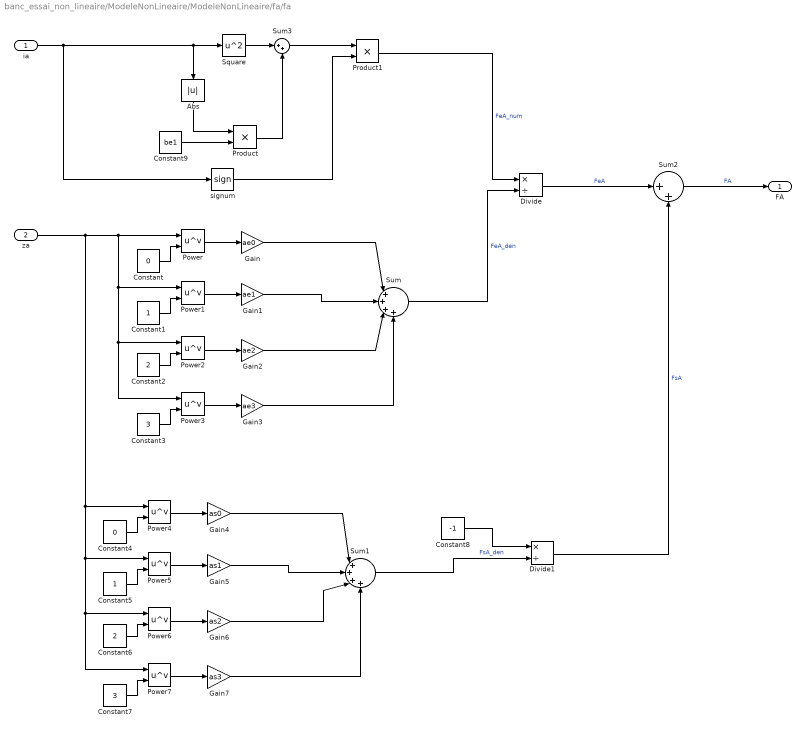
== system banc_essai_non_lineaire/ModeleNonLineaire/ModeleNonLineaire/fa/fa ==
  ia : Inport
  za : Inport  Port=2
  Abs : Abs
  Constant : Constant  Value=0
  Constant1 : Constant
  Constant2 : Constant  Value=2
  Constant3 : Constant  Value=3
  Constant4 : Constant  Value=0
  Constant5 : Constant
  Constant6 : Constant  Value=2
  Constant7 : Constant  Value=3
  Constant8 : Constant  Value=-1
  Constant9 : Constant  Value=be1
  Divide : Product  Inputs=*/
  Divide1 : Product  Inputs=*/
  Gain : Gain  Gain=ae0
  Gain1 : Gain  Gain=ae1
  Gain2 : Gain  Gain=ae2
  Gain3 : Gain  Gain=ae3
  Gain4 : Gain  Gain=as0
  Gain5 : Gain  Gain=as1
  Gain6 : Gain  Gain=as2
  Gain7 : Gain  Gain=as3
  Power{,1..7} (8 alike) : Math  Operator=pow  SaturateOnIntegerOverflow=on
  Product : Product
  Product1 : Product
  Square : Math  Operator=square  SaturateOnIntegerOverflow=on
  Sum : Sum  Inputs=|++++
  Sum1 : Sum  Inputs=|++++
  Sum2 : Sum  Inputs=|++
  Sum3 : Sum  Inputs=|++
  signum : Signum
  FA : Outport
  wires:
  Sum3/1 -> Product1/1
  signum/1 -> Product1/2
  Abs/1 -> Product/1
  ia/1 -> signum/1, Square/1, Abs/1
  Product/1 -> Sum3/2
  Square/1 -> Sum3/1
  Constant9/1 -> Product/2
  Product1/1 -> Divide/1  "FeA_num"
  Sum/1 -> Divide/2  "FeA_den"
  Power/1 -> Gain/1
  Gain2/1 -> Sum/3
  Power1/1 -> Gain1/1
  Gain3/1 -> Sum/4
  Power2/1 -> Gain2/1
  Gain1/1 -> Sum/2
  Gain/1 -> Sum/1
  Power3/1 -> Gain3/1
  Constant2/1 -> Power2/2
  Constant/1 -> Power/2
  Constant3/1 -> Power3/2
  Constant1/1 -> Power1/2
  Divide/1 -> Sum2/1  "FeA"
  Sum1/1 -> Divide1/2  "FsA_den"
  Power4/1 -> Gain4/1
  Gain6/1 -> Sum1/3
  Power5/1 -> Gain5/1
  Gain7/1 -> Sum1/4
  Power6/1 -> Gain6/1
  Gain5/1 -> Sum1/2
  Gain4/1 -> Sum1/1
  Power7/1 -> Gain7/1
  za/1 -> Power7/1, Power6/1, Power5/1, Power4/1, Power3/1, Power2/1, Power1/1, Power/1
  Constant6/1 -> Power6/2
  Constant4/1 -> Power4/2
  Constant7/1 -> Power7/2
  Constant5/1 -> Power5/2
  Constant8/1 -> Divide1/1
  Divide1/1 -> Sum2/2  "FsA"
  Sum2/1 -> FA/1  "FA"

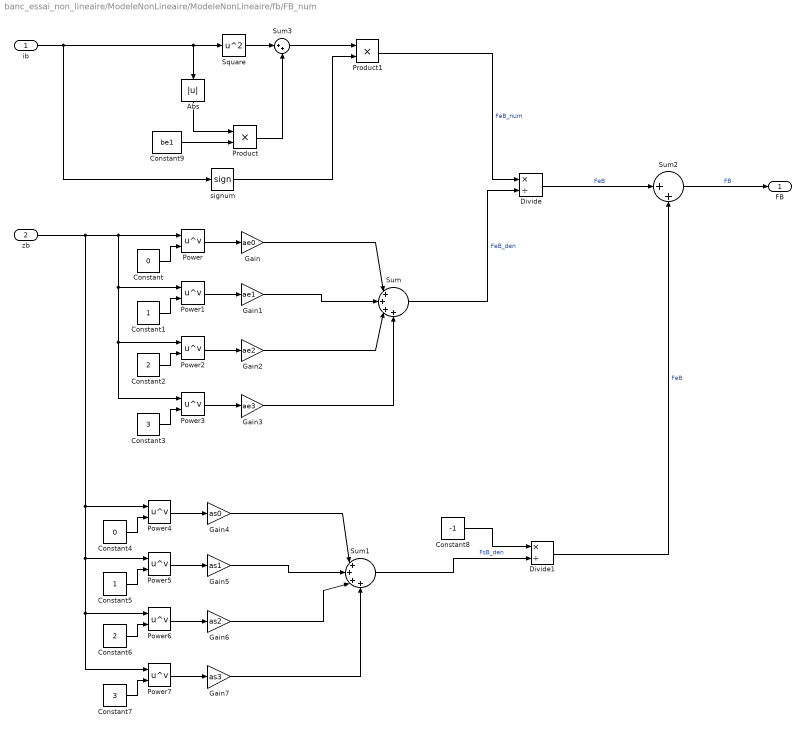
== system banc_essai_non_lineaire/ModeleNonLineaire/ModeleNonLineaire/fb/FB_num ==
  ib : Inport
  zb : Inport  Port=2
  Abs : Abs
  Constant : Constant  Value=0
  Constant1 : Constant
  Constant2 : Constant  Value=2
  Constant3 : Constant  Value=3
  Constant4 : Constant  Value=0
  Constant5 : Constant
  Constant6 : Constant  Value=2
  Constant7 : Constant  Value=3
  Constant8 : Constant  Value=-1
  Constant9 : Constant  Value=be1
  Divide : Product  Inputs=*/
  Divide1 : Product  Inputs=*/
  Gain : Gain  Gain=ae0
  Gain1 : Gain  Gain=ae1
  Gain2 : Gain  Gain=ae2
  Gain3 : Gain  Gain=ae3
  Gain4 : Gain  Gain=as0
  Gain5 : Gain  Gain=as1
  Gain6 : Gain  Gain=as2
  Gain7 : Gain  Gain=as3
  Power{,1..7} (8 alike) : Math  Operator=pow  SaturateOnIntegerOverflow=on
  Product : Product
  Product1 : Product
  Square : Math  Operator=square  SaturateOnIntegerOverflow=on
  Sum : Sum  Inputs=|++++
  Sum1 : Sum  Inputs=|++++
  Sum2 : Sum  Inputs=|++
  Sum3 : Sum  Inputs=|++
  signum : Signum
  FB : Outport
  wires:
  Sum3/1 -> Product1/1
  signum/1 -> Product1/2
  Abs/1 -> Product/1
  ib/1 -> signum/1, Square/1, Abs/1
  Product/1 -> Sum3/2
  Square/1 -> Sum3/1
  Constant9/1 -> Product/2
  Product1/1 -> Divide/1  "FeB_num"
  Sum/1 -> Divide/2  "FeB_den"
  Power/1 -> Gain/1
  Gain2/1 -> Sum/3
  Power1/1 -> Gain1/1
  Gain3/1 -> Sum/4
  Power2/1 -> Gain2/1
  Gain1/1 -> Sum/2
  Gain/1 -> Sum/1
  Power3/1 -> Gain3/1
  Constant2/1 -> Power2/2
  Constant/1 -> Power/2
  Constant3/1 -> Power3/2
  Constant1/1 -> Power1/2
  Divide/1 -> Sum2/1  "FeB"
  Sum1/1 -> Divide1/2  "FsB_den"
  Power4/1 -> Gain4/1
  Gain6/1 -> Sum1/3
  Power5/1 -> Gain5/1
  Gain7/1 -> Sum1/4
  Power6/1 -> Gain6/1
  Gain5/1 -> Sum1/2
  Gain4/1 -> Sum1/1
  Power7/1 -> Gain7/1
  zb/1 -> Power7/1, Power6/1, Power5/1, Power4/1, Power3/1, Power2/1, Power1/1, Power/1
  Constant6/1 -> Power6/2
  Constant4/1 -> Power4/2
  Constant7/1 -> Power7/2
  Constant5/1 -> Power5/2
  Constant8/1 -> Divide1/1
  Divide1/1 -> Sum2/2  "FeB"
  Sum2/1 -> FB/1  "FB"

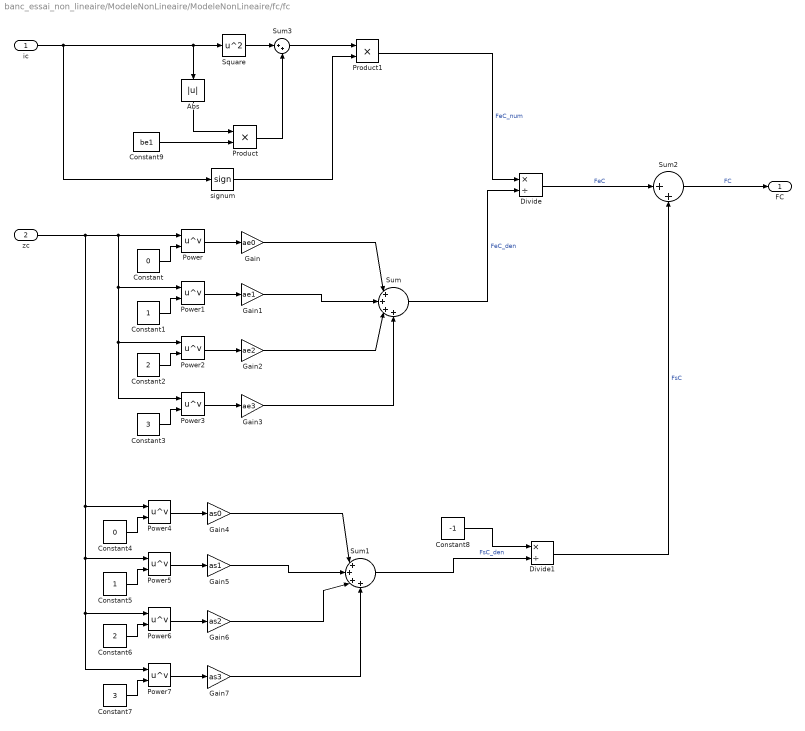
== system banc_essai_non_lineaire/ModeleNonLineaire/ModeleNonLineaire/fc/fc ==
  ic : Inport
  zc : Inport  Port=2
  Abs : Abs
  Constant : Constant  Value=0
  Constant1 : Constant
  Constant2 : Constant  Value=2
  Constant3 : Constant  Value=3
  Constant4 : Constant  Value=0
  Constant5 : Constant
  Constant6 : Constant  Value=2
  Constant7 : Constant  Value=3
  Constant8 : Constant  Value=-1
  Constant9 : Constant  Value=be1
  Divide : Product  Inputs=*/
  Divide1 : Product  Inputs=*/
  Gain : Gain  Gain=ae0
  Gain1 : Gain  Gain=ae1
  Gain2 : Gain  Gain=ae2
  Gain3 : Gain  Gain=ae3
  Gain4 : Gain  Gain=as0
  Gain5 : Gain  Gain=as1
  Gain6 : Gain  Gain=as2
  Gain7 : Gain  Gain=as3
  Power{,1..7} (8 alike) : Math  Operator=pow  SaturateOnIntegerOverflow=on
  Product : Product
  Product1 : Product
  Square : Math  Operator=square  SaturateOnIntegerOverflow=on
  Sum : Sum  Inputs=|++++
  Sum1 : Sum  Inputs=|++++
  Sum2 : Sum  Inputs=|++
  Sum3 : Sum  Inputs=|++
  signum : Signum
  FC : Outport
  wires:
  Sum3/1 -> Product1/1
  signum/1 -> Product1/2
  Abs/1 -> Product/1
  ic/1 -> signum/1, Square/1, Abs/1
  Product/1 -> Sum3/2
  Square/1 -> Sum3/1
  Constant9/1 -> Product/2
  Product1/1 -> Divide/1  "FeC_num"
  Sum/1 -> Divide/2  "FeC_den"
  Power/1 -> Gain/1
  Gain2/1 -> Sum/3
  Power1/1 -> Gain1/1
  Gain3/1 -> Sum/4
  Power2/1 -> Gain2/1
  Gain1/1 -> Sum/2
  Gain/1 -> Sum/1
  Power3/1 -> Gain3/1
  Constant2/1 -> Power2/2
  Constant/1 -> Power/2
  Constant3/1 -> Power3/2
  Constant1/1 -> Power1/2
  Divide/1 -> Sum2/1  "FeC"
  Sum1/1 -> Divide1/2  "FsC_den"
  Power4/1 -> Gain4/1
  Gain6/1 -> Sum1/3
  Power5/1 -> Gain5/1
  Gain7/1 -> Sum1/4
  Power6/1 -> Gain6/1
  Gain5/1 -> Sum1/2
  Gain4/1 -> Sum1/1
  Power7/1 -> Gain7/1
  zc/1 -> Power7/1, Power6/1, Power5/1, Power4/1, Power3/1, Power2/1, Power1/1, Power/1
  Constant6/1 -> Power6/2
  Constant4/1 -> Power4/2
  Constant7/1 -> Power7/2
  Constant5/1 -> Power5/2
  Constant8/1 -> Divide1/1
  Divide1/1 -> Sum2/2  "FsC"
  Sum2/1 -> FC/1  "FC"
